simulink model "lab_otu_pid"  (R2023a)
settings: Solver=VariableStepAuto  StartTime=0.0  StopTime=10  RelTol=1e-3
settings Model: Creator=gnomy  LastModifiedBy=LENOVO

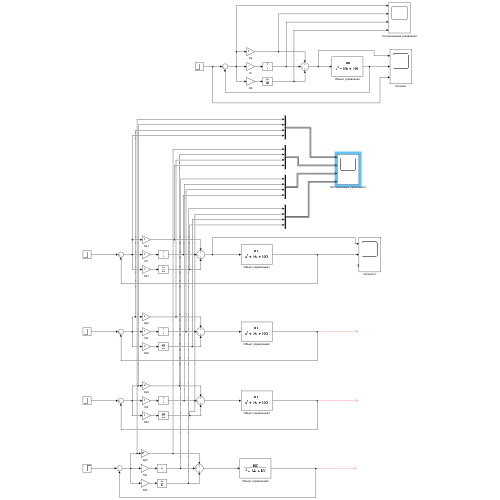
[thumbnail: Simulink's stored preview of the top-level diagram]
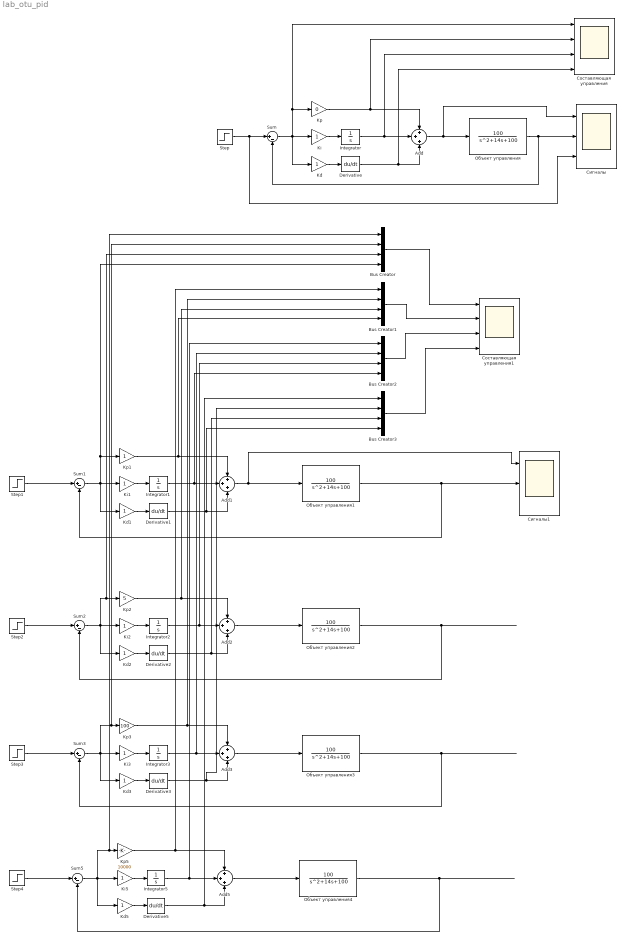
== system lab_otu_pid ==
  Add{,1..3,5} (5 alike) : Sum  Inputs=+++
  Bus Creator{,1..3} (4 alike) : BusCreator  Inputs=4
  Derivative{,1..3,5} (5 alike) : Derivative
  Integrator{,1..3,5} (5 alike) : Integrator
  Kd{,1..3,5} (5 alike) : Gain
  Ki{,1..3,5} (5 alike) : Gain
  Kp : Gain  Gain=0
  Kp1 : Gain
  Kp2 : Gain  Gain=5
  Kp3 : Gain  Gain=100
  Kp5 : Gain  Gain=10000
  Step{,1..4} (5 alike) : Step  SampleTime=0
  Sum{,1..3,5} (5 alike) : Sum  Inputs=|+-
  Объект управления{,1..4} (5 alike) : TransferFcn  Numerator=[100]  Denominator=[1 14 100]
  Сигналы : Scope  NumInputPorts=3
  Сигналы1 : Scope  NumInputPorts=3
  Составляющая управления : Scope  NumInputPorts=4
  Составляющая управления1 : Scope  NumInputPorts=4
  wires:
  Ki/1 -> Integrator/1
  Kd/1 -> Derivative/1
  Kp/1 -> Составляющая управления/2, Add/1
  Integrator/1 -> Составляющая управления/3, Add/2
  Derivative/1 -> Составляющая управления/4, Add/3
  Sum/1 -> Kd/1, Составляющая управления/1, Kp/1, Ki/1
  Add/1 -> Сигналы/1, Объект управления/1
  Step/1 -> Сигналы/3, Sum/1
  Объект управления/1 -> Sum/2, Сигналы/2
  Integrator1/1 -> Bus Creator2/4, Add1/2
  Derivative1/1 -> Bus Creator3/4, Add1/3
  Sum1/1 -> Kd1/1, Bus Creator/4, Kp1/1, Ki1/1
  Kp1/1 -> Bus Creator1/4, Add1/1
  Kd1/1 -> Derivative1/1
  Ki1/1 -> Integrator1/1
  Sum2/1 -> Kd2/1, Bus Creator/3, Kp2/1, Ki2/1
  Kd2/1 -> Derivative2/1
  Ki2/1 -> Integrator2/1
  Kp2/1 -> Bus Creator1/3, Add2/1
  Integrator2/1 -> Bus Creator2/3, Add2/2
  Derivative2/1 -> Bus Creator3/3, Add2/3
  Sum3/1 -> Kd3/1, Bus Creator/2, Kp3/1, Ki3/1
  Kd3/1 -> Derivative3/1
  Ki3/1 -> Integrator3/1
  Kp3/1 -> Add3/1, Bus Creator1/2
  Integrator3/1 -> Bus Creator2/2, Add3/2
  Derivative3/1 -> Bus Creator3/2, Add3/3
  Sum5/1 -> Kd5/1, Bus Creator/1, Kp5/1, Ki5/1
  Kd5/1 -> Derivative5/1
  Ki5/1 -> Integrator5/1
  Kp5/1 -> Bus Creator1/1, Add5/1
  Integrator5/1 -> Bus Creator2/1, Add5/2
  Derivative5/1 -> Bus Creator3/1, Add5/3
  Step1/1 -> Sum1/1
  Объект управления1/1 -> Sum1/2, Сигналы1/2
  Add1/1 -> Объект управления1/1, Сигналы1/1
  Bus Creator/1 -> Составляющая управления1/1
  Bus Creator3/1 -> Составляющая управления1/4
  Bus Creator2/1 -> Составляющая управления1/3
  Bus Creator1/1 -> Составляющая управления1/2
  Add2/1 -> Объект управления2/1
  Объект управления2/1 -> Sum2/2
  Step2/1 -> Sum2/1
  Step3/1 -> Sum3/1
  Step4/1 -> Sum5/1
  Объект управления3/1 -> Sum3/2
  Add3/1 -> Объект управления3/1
  Объект управления4/1 -> Sum5/2
  Add5/1 -> Объект управления4/1
